simulink library "LinkLayer"  (Simulink 7.4)
settings: Solver=ode45  StartTime=0.0  StopTime=10.0  RelTol=1e-3
settings Model: Creator=dread  LastModifiedBy=dread

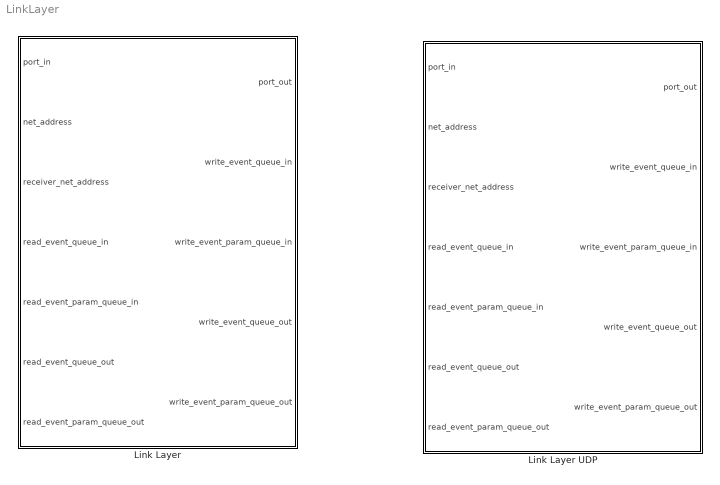
== system LinkLayer ==
  Link Layer : Subsystem  SystemSampleTime=0.1  mask{DelayMin=2, DelayMax=100, MessageLossProbability=0, BufferOverflowPossible=on}
      mask TabNameString: QoS,QoS,QoS,QoS
  Link Layer UDP : Subsystem  SystemSampleTime=0.1  mask{DelayMin=2, DelayMax=100, MessageLossProbability=0}
      mask TabNameString: QoS,QoS,QoS

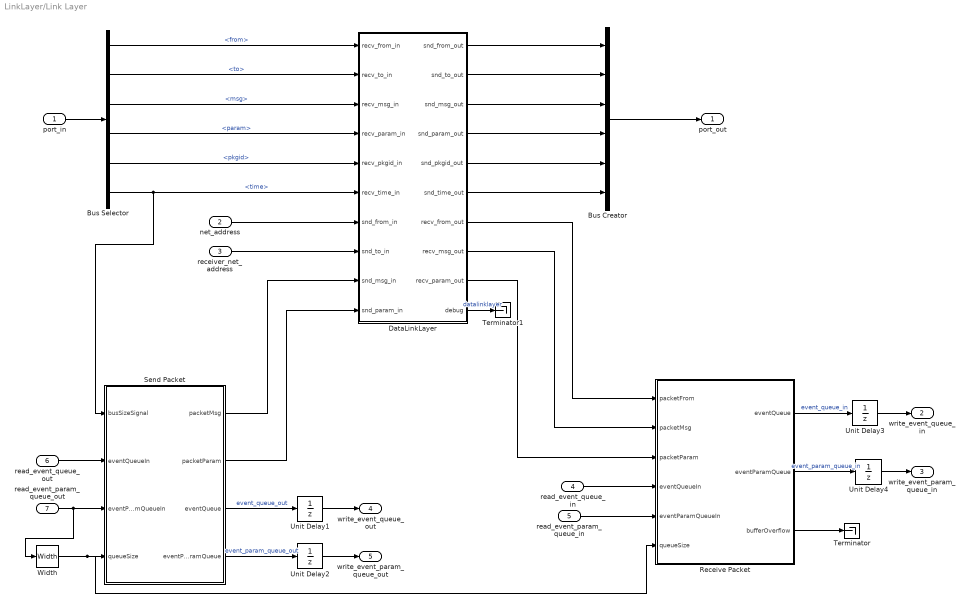
== system LinkLayer/Link Layer ==
  port_in : Inport  UseBusObject=on  OutDataType=fixdt(1, 16)  OutScaling=2^0
      settings: BusObject=PacketBus
  net_address : Inport  Port=2  DataType=uint8  OutDataType=fixdt(1, 16)  OutScaling=2^0  OutDataTypeStr=uint8
  receiver_net_address : Inport  Port=3  DataType=uint8  OutDataType=fixdt(1, 16)  OutScaling=2^0  OutDataTypeStr=uint8
  read_event_queue_in : Inport  Port=4  OutDataType=fixdt(1, 16)  OutScaling=2^0
  read_event_param_queue_in : Inport  Port=5  OutDataType=fixdt(1, 16)  OutScaling=2^0
  read_event_queue_out : Inport  Port=6  OutDataType=fixdt(1, 16)  OutScaling=2^0
  read_event_param_queue_out : Inport  Port=7  OutDataType=fixdt(1, 16)  OutScaling=2^0
  Bus Creator : BusCreator  Inputs=6  UseBusObject=on  NonVirtualBus=on
      settings: BusObject=PacketBus
  Bus Selector : BusSelector  OutputSignals=from,to,msg,param,pkgid,time
  DataLinkLayer : Subsystem
  Receive Packet : Stateflow chart
  Send Packet : Stateflow chart
  Terminator : Terminator
  Terminator1 : Terminator
  Unit Delay{1..4} (4 alike) : UnitDelay  SampleTime=-1
  Width : Width  DataType=uint32
  port_out : Outport  UseBusObject=on  OutDataType=fixdt(1, 16)  OutScaling=2^0
      settings: BusObject=PacketBus
  write_event_queue_in : Outport  Port=2  OutDataType=fixdt(1, 16)  OutScaling=2^0
  write_event_param_queue_in : Outport  Port=3  OutDataType=fixdt(1, 16)  OutScaling=2^0
  write_event_queue_out : Outport  Port=4  OutDataType=fixdt(1, 16)  OutScaling=2^0
  write_event_param_queue_out : Outport  Port=5  OutDataType=fixdt(1, 16)  OutScaling=2^0
  wires:
  Receive Packet/2(eventParamQueue) -> Unit Delay4/1  "event_param_queue_in"
  Receive Packet/1(eventQueue) -> Unit Delay3/1  "event_queue_in"
  Send Packet/4(eventParamQueue) -> Unit Delay2/1  "event_param_queue_out"
  Send Packet/3(eventQueue) -> Unit Delay1/1  "event_queue_out"
  read_event_queue_out/1 -> Send Packet/2(eventQueueIn)
  net_address/1 -> DataLinkLayer/7(snd_from_in)
  Send Packet/1(packetMsg) -> DataLinkLayer/9(snd_msg_in)
  DataLinkLayer/9(recv_param_out) -> Receive Packet/3(packetParam)
  DataLinkLayer/8(recv_msg_out) -> Receive Packet/2(packetMsg)
  DataLinkLayer/7(recv_from_out) -> Receive Packet/1(packetFrom)
  Bus Selector/3 -> DataLinkLayer/3(recv_msg_in)  "<msg>"
  Bus Selector/5 -> DataLinkLayer/5(recv_pkgid_in)  "<pkgid>"
  Bus Selector/6 -> Send Packet/1(busSizeSignal), DataLinkLayer/6(recv_time_in)  "<time>"
  port_in/1 -> Bus Selector/1
  Bus Creator/1 -> port_out/1
  Bus Selector/2 -> DataLinkLayer/2(recv_to_in)  "<to>"
  Bus Selector/1 -> DataLinkLayer/1(recv_from_in)  "<from>"
  Send Packet/2(packetParam) -> DataLinkLayer/10(snd_param_in)
  Bus Selector/4 -> DataLinkLayer/4(recv_param_in)  "<param>"
  read_event_queue_in/1 -> Receive Packet/4(eventQueueIn)
  read_event_param_queue_in/1 -> Receive Packet/5(eventParamQueueIn)
  read_event_param_queue_out/1 -> Send Packet/3(eventParamQueueIn), Width/1
  DataLinkLayer/1(snd_from_out) -> Bus Creator/1
  DataLinkLayer/2(snd_to_out) -> Bus Creator/2
  DataLinkLayer/3(snd_msg_out) -> Bus Creator/3
  DataLinkLayer/4(snd_param_out) -> Bus Creator/4
  DataLinkLayer/5(snd_pkgid_out) -> Bus Creator/5
  DataLinkLayer/6(snd_time_out) -> Bus Creator/6
  Receive Packet/3(bufferOverflow) -> Terminator/1
  Unit Delay1/1 -> write_event_queue_out/1
  Unit Delay2/1 -> write_event_param_queue_out/1
  Unit Delay3/1 -> write_event_queue_in/1
  Unit Delay4/1 -> write_event_param_queue_in/1
  receiver_net_address/1 -> DataLinkLayer/8(snd_to_in)
  Width/1 -> Receive Packet/6(queueSize), Send Packet/4(queueSize)
  DataLinkLayer/10(debug) -> Terminator1/1  "datalinklayer"

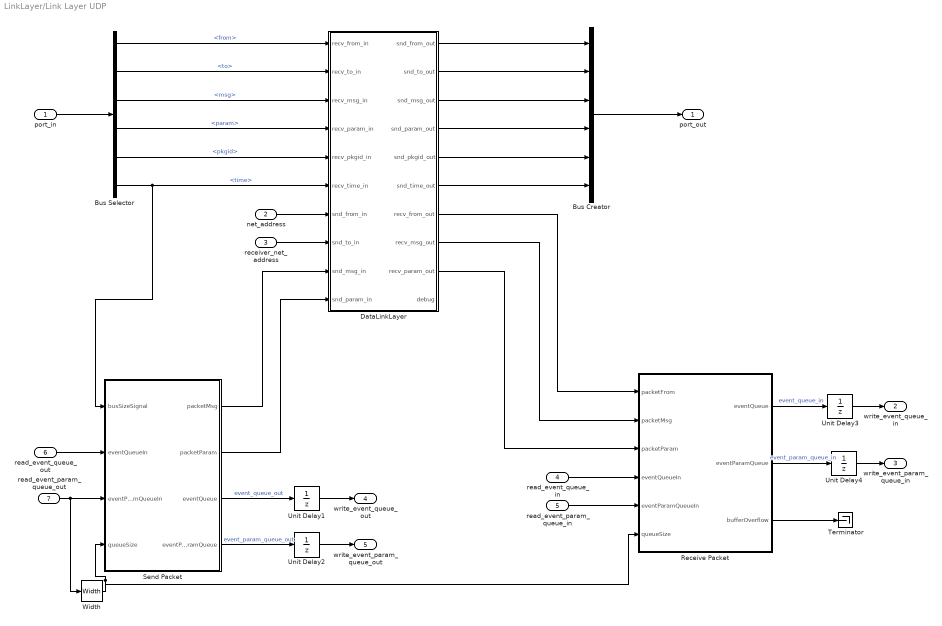
== system LinkLayer/Link Layer UDP ==
  port_in : Inport  UseBusObject=on  OutDataType=fixdt(1, 16)  OutScaling=2^0
      settings: BusObject=PacketBus
  net_address : Inport  Port=2  DataType=uint8  OutDataType=fixdt(1, 16)  OutScaling=2^0  OutDataTypeStr=uint8
  receiver_net_address : Inport  Port=3  DataType=uint8  OutDataType=fixdt(1, 16)  OutScaling=2^0  OutDataTypeStr=uint8
  read_event_queue_in : Inport  Port=4  OutDataType=fixdt(1, 16)  OutScaling=2^0
  read_event_param_queue_in : Inport  Port=5  OutDataType=fixdt(1, 16)  OutScaling=2^0
  read_event_queue_out : Inport  Port=6  OutDataType=fixdt(1, 16)  OutScaling=2^0
  read_event_param_queue_out : Inport  Port=7  OutDataType=fixdt(1, 16)  OutScaling=2^0
  Bus Creator : BusCreator  Inputs=6  UseBusObject=on
      settings: BusObject=PacketBus
  Bus Selector : BusSelector  OutputSignals=from,to,msg,param,pkgid,time
  DataLinkLayer : Subsystem
  Receive Packet : Stateflow chart
  Send Packet : Stateflow chart
  Terminator : Terminator
  Unit Delay{1..4} (4 alike) : UnitDelay  SampleTime=-1
  Width : Width  DataType=uint32
  port_out : Outport  UseBusObject=on  OutDataType=fixdt(1, 16)  OutScaling=2^0
      settings: BusObject=PacketBus
  write_event_queue_in : Outport  Port=2  OutDataType=fixdt(1, 16)  OutScaling=2^0
  write_event_param_queue_in : Outport  Port=3  OutDataType=fixdt(1, 16)  OutScaling=2^0
  write_event_queue_out : Outport  Port=4  OutDataType=fixdt(1, 16)  OutScaling=2^0
  write_event_param_queue_out : Outport  Port=5  OutDataType=fixdt(1, 16)  OutScaling=2^0
  wires:
  net_address/1 -> DataLinkLayer/7(snd_from_in)
  Send Packet/1(packetMsg) -> DataLinkLayer/9(snd_msg_in)
  DataLinkLayer/9(recv_param_out) -> Receive Packet/3(packetParam)
  DataLinkLayer/8(recv_msg_out) -> Receive Packet/2(packetMsg)
  DataLinkLayer/7(recv_from_out) -> Receive Packet/1(packetFrom)
  Bus Selector/3 -> DataLinkLayer/3(recv_msg_in)  "<msg>"
  Bus Selector/5 -> DataLinkLayer/5(recv_pkgid_in)  "<pkgid>"
  Bus Selector/6 -> Send Packet/1(busSizeSignal), DataLinkLayer/6(recv_time_in)  "<time>"
  port_in/1 -> Bus Selector/1
  Bus Creator/1 -> port_out/1
  Bus Selector/2 -> DataLinkLayer/2(recv_to_in)  "<to>"
  Bus Selector/1 -> DataLinkLayer/1(recv_from_in)  "<from>"
  Send Packet/2(packetParam) -> DataLinkLayer/10(snd_param_in)
  Bus Selector/4 -> DataLinkLayer/4(recv_param_in)  "<param>"
  DataLinkLayer/1(snd_from_out) -> Bus Creator/1
  DataLinkLayer/2(snd_to_out) -> Bus Creator/2
  DataLinkLayer/3(snd_msg_out) -> Bus Creator/3
  DataLinkLayer/4(snd_param_out) -> Bus Creator/4
  DataLinkLayer/5(snd_pkgid_out) -> Bus Creator/5
  DataLinkLayer/6(snd_time_out) -> Bus Creator/6
  Receive Packet/2(eventParamQueue) -> Unit Delay4/1  "event_param_queue_in"
  Receive Packet/1(eventQueue) -> Unit Delay3/1  "event_queue_in"
  Unit Delay3/1 -> write_event_queue_in/1
  Unit Delay4/1 -> write_event_param_queue_in/1
  Receive Packet/3(bufferOverflow) -> Terminator/1
  Send Packet/4(eventParamQueue) -> Unit Delay2/1  "event_param_queue_out"
  Send Packet/3(eventQueue) -> Unit Delay1/1  "event_queue_out"
  Unit Delay1/1 -> write_event_queue_out/1
  Unit Delay2/1 -> write_event_param_queue_out/1
  receiver_net_address/1 -> DataLinkLayer/8(snd_to_in)
  read_event_queue_in/1 -> Receive Packet/4(eventQueueIn)
  read_event_param_queue_in/1 -> Receive Packet/5(eventParamQueueIn)
  read_event_queue_out/1 -> Send Packet/2(eventQueueIn)
  read_event_param_queue_out/1 -> Send Packet/3(eventParamQueueIn), Width/1
  Width/1 -> Send Packet/4(queueSize), Receive Packet/6(queueSize)

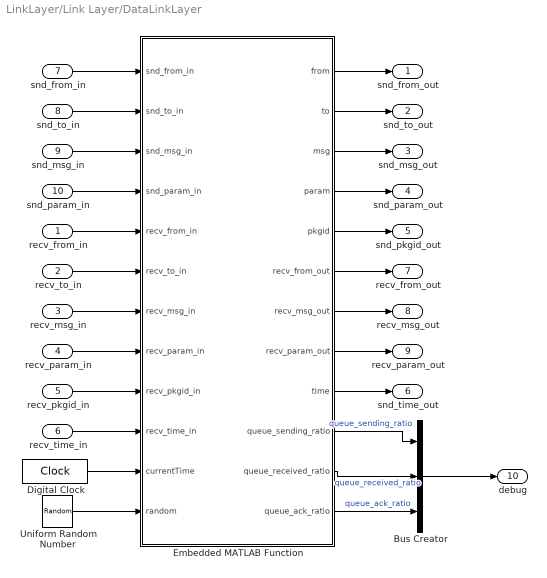
== system LinkLayer/Link Layer/DataLinkLayer ==
  recv_from_in : Inport  DataType=uint8  OutDataType=fixdt(1, 16)  OutScaling=2^0  OutDataTypeStr=uint8
  recv_to_in : Inport  Port=2  DataType=uint8  OutDataType=fixdt(1, 16)  OutScaling=2^0  OutDataTypeStr=uint8
  recv_msg_in : Inport  Port=3  DataType=uint16  OutDataType=fixdt(1, 16)  OutScaling=2^0  OutDataTypeStr=uint16
  recv_param_in : Inport  Port=4  DataType=double  OutDataType=fixdt(1, 16)  OutScaling=2^0  OutDataTypeStr=double
  recv_pkgid_in : Inport  Port=5  DataType=uint32  OutDataType=fixdt(1, 16)  OutScaling=2^0  OutDataTypeStr=uint32
  recv_time_in : Inport  Port=6  DataType=double  OutDataType=fixdt(1, 16)  OutScaling=2^0  OutDataTypeStr=double
  snd_from_in : Inport  Port=7  DataType=uint8  OutDataType=fixdt(1, 16)  OutScaling=2^0  OutDataTypeStr=uint8
  snd_to_in : Inport  Port=8  DataType=uint8  OutDataType=fixdt(1, 16)  OutScaling=2^0  OutDataTypeStr=uint8
  snd_msg_in : Inport  Port=9  DataType=uint16  OutDataType=fixdt(1, 16)  OutScaling=2^0  OutDataTypeStr=uint16
  snd_param_in : Inport  Port=10  DataType=double  OutDataType=fixdt(1, 16)  OutScaling=2^0  OutDataTypeStr=double
  Bus Creator : BusCreator  Inputs=3
  Digital Clock : DigitalClock  SampleTime=0.001
  Embedded MATLAB Function : Stateflow chart  TreatAsAtomicUnit=on
  Uniform Random Number : UniformRandomNumber  Minimum=0  Maximum=100  SampleTime=0.001
  snd_from_out : Outport  DataType=uint8  OutDataType=fixdt(1, 16)  OutScaling=2^0  OutDataTypeStr=uint8
  snd_to_out : Outport  Port=2  DataType=uint8  OutDataType=fixdt(1, 16)  OutScaling=2^0  OutDataTypeStr=uint8
  snd_msg_out : Outport  Port=3  DataType=uint16  OutDataType=fixdt(1, 16)  OutScaling=2^0  OutDataTypeStr=uint16
  snd_param_out : Outport  Port=4  DataType=double  OutDataType=fixdt(1, 16)  OutScaling=2^0  OutDataTypeStr=double
  snd_pkgid_out : Outport  Port=5  DataType=uint32  OutDataType=fixdt(1, 16)  OutScaling=2^0  OutDataTypeStr=uint32
  snd_time_out : Outport  Port=6  DataType=double  OutDataType=fixdt(1, 16)  OutScaling=2^0  OutDataTypeStr=double
  recv_from_out : Outport  Port=7  DataType=uint8  OutDataType=fixdt(1, 16)  OutScaling=2^0  OutDataTypeStr=uint8
  recv_msg_out : Outport  Port=8  DataType=uint16  OutDataType=fixdt(1, 16)  OutScaling=2^0  OutDataTypeStr=uint16
  recv_param_out : Outport  Port=9  DataType=double  OutDataType=fixdt(1, 16)  OutScaling=2^0  OutDataTypeStr=double
  debug : Outport  Port=10  OutDataType=fixdt(1, 16)  OutScaling=2^0
  wires:
  Embedded MATLAB Function/9(time) -> snd_time_out/1
  recv_time_in/1 -> Embedded MATLAB Function/10(recv_time_in)
  recv_pkgid_in/1 -> Embedded MATLAB Function/9(recv_pkgid_in)
  recv_param_in/1 -> Embedded MATLAB Function/8(recv_param_in)
  recv_msg_in/1 -> Embedded MATLAB Function/7(recv_msg_in)
  recv_to_in/1 -> Embedded MATLAB Function/6(recv_to_in)
  recv_from_in/1 -> Embedded MATLAB Function/5(recv_from_in)
  Embedded MATLAB Function/8(recv_param_out) -> recv_param_out/1
  Embedded MATLAB Function/7(recv_msg_out) -> recv_msg_out/1
  Embedded MATLAB Function/6(recv_from_out) -> recv_from_out/1
  snd_to_in/1 -> Embedded MATLAB Function/2(snd_to_in)
  snd_from_in/1 -> Embedded MATLAB Function/1(snd_from_in)
  snd_param_in/1 -> Embedded MATLAB Function/4(snd_param_in)
  snd_msg_in/1 -> Embedded MATLAB Function/3(snd_msg_in)
  Embedded MATLAB Function/5(pkgid) -> snd_pkgid_out/1
  Embedded MATLAB Function/4(param) -> snd_param_out/1
  Embedded MATLAB Function/3(msg) -> snd_msg_out/1
  Embedded MATLAB Function/2(to) -> snd_to_out/1
  Embedded MATLAB Function/1(from) -> snd_from_out/1
  Bus Creator/1 -> debug/1
  Embedded MATLAB Function/10(queue_sending_ratio) -> Bus Creator/1  "queue_sending_ratio"
  Embedded MATLAB Function/11(queue_received_ratio) -> Bus Creator/2  "queue_received_ratio"
  Embedded MATLAB Function/12(queue_ack_ratio) -> Bus Creator/3  "queue_ack_ratio"
  Digital Clock/1 -> Embedded MATLAB Function/11(currentTime)
  Uniform Random Number/1 -> Embedded MATLAB Function/12(random)

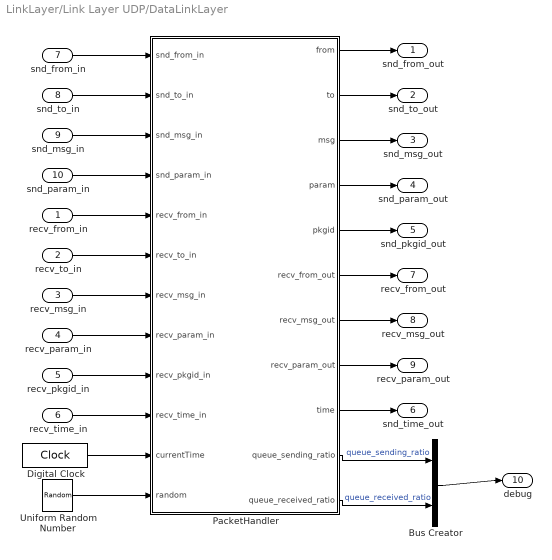
== system LinkLayer/Link Layer UDP/DataLinkLayer ==
  recv_from_in : Inport  DataType=uint8  OutDataType=fixdt(1, 16)  OutScaling=2^0  OutDataTypeStr=uint8
  recv_to_in : Inport  Port=2  DataType=uint8  OutDataType=fixdt(1, 16)  OutScaling=2^0  OutDataTypeStr=uint8
  recv_msg_in : Inport  Port=3  DataType=uint16  OutDataType=fixdt(1, 16)  OutScaling=2^0  OutDataTypeStr=uint16
  recv_param_in : Inport  Port=4  DataType=double  OutDataType=fixdt(1, 16)  OutScaling=2^0  OutDataTypeStr=double
  recv_pkgid_in : Inport  Port=5  DataType=uint32  OutDataType=fixdt(1, 16)  OutScaling=2^0  OutDataTypeStr=uint32
  recv_time_in : Inport  Port=6  DataType=double  OutDataType=fixdt(1, 16)  OutScaling=2^0  OutDataTypeStr=double
  snd_from_in : Inport  Port=7  DataType=uint8  OutDataType=fixdt(1, 16)  OutScaling=2^0  OutDataTypeStr=uint8
  snd_to_in : Inport  Port=8  DataType=uint8  OutDataType=fixdt(1, 16)  OutScaling=2^0  OutDataTypeStr=uint8
  snd_msg_in : Inport  Port=9  DataType=uint16  OutDataType=fixdt(1, 16)  OutScaling=2^0  OutDataTypeStr=uint16
  snd_param_in : Inport  Port=10  DataType=double  OutDataType=fixdt(1, 16)  OutScaling=2^0  OutDataTypeStr=double
  Bus Creator : BusCreator  Inputs=2
  Digital Clock : DigitalClock  SampleTime=-1
  PacketHandler : Stateflow chart  TreatAsAtomicUnit=on
  Uniform Random Number : UniformRandomNumber  Minimum=0  Maximum=100  SampleTime=0.001
  snd_from_out : Outport  DataType=uint8  OutDataType=fixdt(1, 16)  OutScaling=2^0  OutDataTypeStr=uint8
  snd_to_out : Outport  Port=2  DataType=uint8  OutDataType=fixdt(1, 16)  OutScaling=2^0  OutDataTypeStr=uint8
  snd_msg_out : Outport  Port=3  DataType=uint16  OutDataType=fixdt(1, 16)  OutScaling=2^0  OutDataTypeStr=uint16
  snd_param_out : Outport  Port=4  DataType=double  OutDataType=fixdt(1, 16)  OutScaling=2^0  OutDataTypeStr=double
  snd_pkgid_out : Outport  Port=5  DataType=uint32  OutDataType=fixdt(1, 16)  OutScaling=2^0  OutDataTypeStr=uint32
  snd_time_out : Outport  Port=6  DataType=double  OutDataType=fixdt(1, 16)  OutScaling=2^0  OutDataTypeStr=double
  recv_from_out : Outport  Port=7  DataType=uint8  OutDataType=fixdt(1, 16)  OutScaling=2^0  OutDataTypeStr=uint8
  recv_msg_out : Outport  Port=8  DataType=uint16  OutDataType=fixdt(1, 16)  OutScaling=2^0  OutDataTypeStr=uint16
  recv_param_out : Outport  Port=9  DataType=double  OutDataType=fixdt(1, 16)  OutScaling=2^0  OutDataTypeStr=double
  debug : Outport  Port=10  OutDataType=fixdt(1, 16)  OutScaling=2^0
  wires:
  PacketHandler/9(time) -> snd_time_out/1
  recv_time_in/1 -> PacketHandler/10(recv_time_in)
  recv_pkgid_in/1 -> PacketHandler/9(recv_pkgid_in)
  recv_param_in/1 -> PacketHandler/8(recv_param_in)
  recv_msg_in/1 -> PacketHandler/7(recv_msg_in)
  recv_to_in/1 -> PacketHandler/6(recv_to_in)
  recv_from_in/1 -> PacketHandler/5(recv_from_in)
  PacketHandler/8(recv_param_out) -> recv_param_out/1
  PacketHandler/7(recv_msg_out) -> recv_msg_out/1
  PacketHandler/6(recv_from_out) -> recv_from_out/1
  snd_to_in/1 -> PacketHandler/2(snd_to_in)
  snd_from_in/1 -> PacketHandler/1(snd_from_in)
  snd_param_in/1 -> PacketHandler/4(snd_param_in)
  snd_msg_in/1 -> PacketHandler/3(snd_msg_in)
  PacketHandler/5(pkgid) -> snd_pkgid_out/1
  PacketHandler/4(param) -> snd_param_out/1
  PacketHandler/3(msg) -> snd_msg_out/1
  PacketHandler/2(to) -> snd_to_out/1
  PacketHandler/1(from) -> snd_from_out/1
  Bus Creator/1 -> debug/1
  PacketHandler/10(queue_sending_ratio) -> Bus Creator/1  "queue_sending_ratio"
  PacketHandler/11(queue_received_ratio) -> Bus Creator/2  "queue_received_ratio"
  Digital Clock/1 -> PacketHandler/11(currentTime)
  Uniform Random Number/1 -> PacketHandler/12(random)

== matlab function Link Layer/Receive Packet ==
  settings: updateMethod=DISCRETE  sampleTime=0.001
  data: packetFrom input double; packetMsg input double; packetParam input double; eventQueueIn input uint8; eventParamQueueIn input double; eventQueue output uint8; eventParamQueue output double; bufferOverflow output boolean; queueSize input uint32
function [eventQueue, eventParamQueue, bufferOverflow] = receivePacket(packetFrom, packetMsg, packetParam, eventQueueIn, eventParamQueueIn, queueSize)
%#eml
% This function receives packets and adds them to the event queue.
% A packet consists of a source, a message and an optional parameter for 
% the message. Source and message are contained at position 1 and 2 in the 
% eventQueue. Because of the different data type the parameter has his own 
% queue eventParamQueue.

%Constants
SOURCE = 2;
MESSAGE = 1;
BUS_SIZE = numel(packetFrom);
QUEUE_SIZE = queueSize;

%Init
eventQueue = eventQueueIn;
eventParamQueue = eventParamQueueIn;
bufferOverflow = false;

%New incoming packet
for i = 1:BUS_SIZE
    if packetFrom(i) ~= 0 
        bufferOverflow = true;
        %Add it to the incoming event Queue
        for j = 1:QUEUE_SIZE
            %Search for an empty place
            if eventQueue(j,SOURCE) == 0
                eventQueue(j,SOURCE)    = packetFrom(i);
                eventQueue(j,MESSAGE)   = packetMsg(i);
                eventParamQueue(j)      = packetParam(i);
                bufferOverflow = false;
                break;
            end
        end        
    else
        break;
    end
end

== matlab function Link Layer/Send Packet ==
  settings: updateMethod=DISCRETE  sampleTime=0.001
  data: busSizeSignal input double; packetMsg output double; packetParam output double; eventQueue output uint8; eventParamQueue output double; eventQueueIn input uint8; eventParamQueueIn input double; queueSize input uint32
function [packetMsg, packetParam, eventQueue, eventParamQueue] = sendPacket(busSizeSignal, eventQueueIn, eventParamQueueIn, queueSize)
%#eml

% This function creates packets from the event queue. A packet consists
% of a destination, a message and an optional parameter for the message.
% Destination and message are contained at position 1 and 2 in the 
% eventQueue. Because of the different data type the parameter has his own 
% queue eventParamQueue.

%Constants
DESTINATION = 2;
MESSAGE = 1;
QUEUE_SIZE = queueSize;

busSize = numel(busSizeSignal);

%Init
eventQueue = eventQueueIn;
eventParamQueue = eventParamQueueIn;
packetMsg = zeros(1,busSize,'uint16');
packetParam = zeros(1,busSize,'double');

%There is an event in the queue
for i = 1:busSize   
    if eventQueue(1,DESTINATION) ~= 0 || eventQueue(1,MESSAGE) ~= 0
        %Create packet from the firs entry in the queue
        packetMsg(i)   = uint16(eventQueue(1,MESSAGE));
        packetParam(i) = eventParamQueue(1);
        %Remove the event from the queue
        for j=1:QUEUE_SIZE - 1
            eventQueue(j,DESTINATION)   = eventQueue(j+1,DESTINATION);
            eventQueue(j,MESSAGE)       = eventQueue(j+1,MESSAGE);
            eventParamQueue(j)          = eventParamQueue(j+1);
        end
        %Set last element to zero
        eventQueue(QUEUE_SIZE,DESTINATION)  = 0;
        eventQueue(QUEUE_SIZE,MESSAGE)      = 0;
        eventParamQueue(QUEUE_SIZE)    = 0;
    else
        break;
    end
end

== matlab function Link Layer UDP/DataLinkLayer/PacketHandler ==
  settings: updateMethod=DISCRETE
  data: snd_from_in input double; snd_to_in input double; snd_msg_in input double; snd_param_in input double; from output double; to output double; msg output double; param output double; pkgid output double; recv_from_in input double; recv_to_in input double; recv_msg_in input double; recv_param_in input double; recv_pkgid_in input uint32; recv_from_out output double; recv_msg_out output double; recv_param_out output double; recv_time_in input double; time output double; currentTime input double; queue_sending_ratio output double; queue_received_ratio output double; DelayMin parameter uint32; DelayMax parameter uint32; MessageLossProbability parameter uint32; random input double
function [from, to, msg, param, pkgid, recv_from_out, recv_msg_out, recv_param_out, time, queue_sending_ratio, queue_received_ratio] = packetHandler(snd_from_in, snd_to_in, snd_msg_in, snd_param_in, recv_from_in, recv_to_in, recv_msg_in, recv_param_in, recv_pkgid_in, recv_time_in, currentTime, DelayMin, DelayMax, MessageLossProbability, random)
%#eml
eml.extrinsic('warning', 'disp', 'fprintf');

%Constants
BUS_SIZE =  1;%numel(snd_from_in);
QUEUE_SIZE_SENDING = 10 * BUS_SIZE;
QUEUE_SIZE_RECEIVED = 10 *BUS_SIZE;
SAMPLE_TIME = 0.001;
PHYSICAL_DELAY = 2;

%Constraints
if DelayMin < 2
    DelayMin = uint32(2);
end

%Time to delay each outgoing packet
assert(DelayMin >= PHYSICAL_DELAY);
delay_time =  double(DelayMin - PHYSICAL_DELAY) * SAMPLE_TIME;

%Init
from    = zeros(1,BUS_SIZE,'uint8');
to      = zeros(1,BUS_SIZE,'uint8');
msg     = zeros(1,BUS_SIZE,'uint16');
param   = zeros(1,BUS_SIZE,'double');
pkgid   = zeros(1,BUS_SIZE,'uint32');
time    = zeros(1,BUS_SIZE,'double');
 
recv_from_out    = zeros(1,BUS_SIZE,'uint8');
recv_msg_out     = zeros(1,BUS_SIZE,'uint16');
recv_param_out   = zeros(1,BUS_SIZE,'double');


recv_in = bus(recv_from_in, recv_to_in, recv_msg_in, recv_param_in, recv_pkgid_in, recv_time_in, BUS_SIZE);



%Persistent variables
persistent sendingQueue receivedQueue lastPkgid

if isempty(lastPkgid)
    lastPkgid = uint32(0);
end

if isempty(sendingQueue)
    sendingQueue = repmat(packet(0,0,0,0,0,0), 1, QUEUE_SIZE_SENDING);
end


if isempty(receivedQueue)
    receivedQueue = repmat(packet(0, 0, 0, 0, 0, 0), 1, QUEUE_SIZE_RECEIVED);
end

%compute stats
queue_sending_ratio = queueNumElements(sendingQueue)/QUEUE_SIZE_SENDING;
queue_received_ratio = queueNumElements(receivedQueue)/QUEUE_SIZE_RECEIVED;

%Step 1: Check for a new outgoing packet
for i = 1:BUS_SIZE    
    if snd_msg_in(i) ~= 0
        lastPkgid = lastPkgid +1;
        outgoing = packet(snd_from_in, snd_to_in(i), snd_msg_in(i), snd_param_in(i), lastPkgid, currentTime);

        %Add packet so the outgoing queue
        sendingQueue = enqueue(sendingQueue, outgoing); 
    end
end
    
%Step 2: Check for a new incoming packet
for i = 1:length(recv_in)
    incoming = packet(recv_in(i).from, recv_in(i).to, recv_in(i).msg, recv_in(i).param, recv_in(i).pkgid, recv_in(i).time);
    if incoming.from ~= 0 && incoming.to == snd_from_in && ~dropPacket(incoming, MessageLossProbability, random)
        
        %Check if max_delay is valid
        if incoming.time + (double(DelayMax) * SAMPLE_TIME) < currentTime
            %Exceeded max delay. Drop packet.
            continue;
        end

        %save packet
        receivedQueue = enqueue(receivedQueue, incoming); 
    end
end

%Step 3: Forward incoming packet
for i = 1:BUS_SIZE
    if receivedQueue(1).from ~= 0
        recv_from_out(i)    = receivedQueue(1).from;
        recv_msg_out(i)     = receivedQueue(1).msg;
        recv_param_out(i)   = receivedQueue(1).param;
        receivedQueue = dequeue(receivedQueue,1);
    else
        break;
    end
end


%Step 4: Send outgoing packet
for i = 1:BUS_SIZE
    if sendingQueue(1).to ~= 0  && minDelayExpired(sendingQueue(1), currentTime, delay_time) %Respect minimum delay
        from(i)    = sendingQueue(1).from;
        to(i)      = sendingQueue(1).to;
        msg(i)     = sendingQueue(1).msg;
        param(i)   = sendingQueue(1).param;
        pkgid(i)   = sendingQueue(1).pkgid;
        time(i)    = sendingQueue(1).time;

        %remove packet from sending queue
        sendingQueue = dequeue(sendingQueue, 1);    
    else
        break;
    end
end


%%%%%%%%%%%%%%%%%%%%%%%%%%%%%%%%%%%%%%%%%%%%%%%%%%%%%%%%%%%%%%%%%%%%%%%%%%%
%%                          H E L P E R
%%%%%%%%%%%%%%%%%%%%%%%%%%%%%%%%%%%%%%%%%%%%%%%%%%%%%%%%%%%%%%%%%%%%%%%%%%%

function p = packet(from, to, msg, param, pkgid, time)
%#eml
%Defines a packet
p = struct('from', uint8(from),'to', uint8(to),'msg', uint16(msg),'param', double(param),'pkgid', uint32(pkgid), 'time', double(time));

function bus = bus(from, to, msg, param, pkgid, time, size) %emp
%Create an empty bus
bus = repmat(packet(0,0,0,0,0,0), 1, size);
for i=1:size
    bus(i) = packet(from(i), to(i), msg(i), param(i), pkgid(i), time(i));
end


function queue = enqueue(queue, packet)
%#eml
eml.extrinsic('warning', 'sprintf');
for i = 1:length(queue)
    if queue(i).to == 0
        queue(i) = packet;
        return;
    end
end
warning('DataLinkLayer:enqueue', 'DataLinkLayer Buffer overflow. Dropping packet  %3u: %u->%u :%3u (%.1f) @%.2f', packet.pkgid, packet.from, packet.to, packet.msg, packet.param, packet.time);

function queue = dequeue(queue, index)
%#eml
assert(index <= length(queue))
for i=index:length(queue)-1;
    queue(i) = queue(i+1);
end
queue(length(queue)) = packet(0,0,0,0,0,0);

function num = queueNumElements(queue)
%#eml
num = 0;
for i = 1:length(queue)
    if queue(i).to ~= uint8(0)
        num = num+1;
    end
end    

function packetString = toString(packet) %#eml
eml.extrinsic('sprintf');
packetString = sprintf('%3u: %u->%u :%3u (%.2f) @%.3f', packet.pkgid, packet.from, packet.to, packet.msg, packet.param, packet.time);

%Wheter the packet is ready to fire or not.
function expired = minDelayExpired(packet, current_time, delay_time) %eml
eml.extrinsic('warning');
expired = (packet.time + delay_time) <= current_time;

%Drop message with a given probability
function drop = dropPacket(p, probability, random) %eml
drop = random < probability;

== matlab function Link Layer/DataLinkLayer/Embedded MATLAB Function ==
  settings: updateMethod=DISCRETE  sampleTime=0.001
  data: snd_from_in input double; snd_to_in input double; snd_msg_in input double; snd_param_in input double; from output double; to output double; msg output double; param output double; pkgid output double; recv_from_in input double; recv_to_in input double; recv_msg_in input double; recv_param_in input double; recv_pkgid_in input uint32; recv_from_out output double; recv_msg_out output double; recv_param_out output double; recv_time_in input double; time output double; currentTime input double; queue_sending_ratio output double; queue_received_ratio output double; queue_ack_ratio output double; DelayMin parameter uint32; DelayMax parameter uint32; BufferOverflowPossible parameter boolean; MessageLossProbability parameter uint32; random input double
function [from, to, msg, param, pkgid, recv_from_out, recv_msg_out, recv_param_out, time, queue_sending_ratio, queue_received_ratio, queue_ack_ratio] = ackHandler(snd_from_in, snd_to_in, snd_msg_in, snd_param_in, recv_from_in, recv_to_in, recv_msg_in, recv_param_in, recv_pkgid_in, recv_time_in, currentTime, DelayMin, DelayMax, BufferOverflowPossible, MessageLossProbability, random)
%#eml
eml.extrinsic('warning', 'disp', 'fprintf', 'error');

%Constants
SAMPLE_TIME = 0.001;
BUS_SIZE =  numel(snd_msg_in);
MSG_ACK         = 255;
QUEUE_SIZE_SENDING = 10 * BUS_SIZE;
QUEUE_SIZE_ACK  = 10* BUS_SIZE;
QUEUE_SIZE_RECEIVED = 10 *BUS_SIZE;
QUEUE_SIZE_INORDER = 10* BUS_SIZE;

PHYSICAL_DELAY = 2;

%Constraints
if DelayMin < PHYSICAL_DELAY
    DelayMin = uint32(PHYSICAL_DELAY);
end

DELAY_MIN_TIME = double(DelayMin) * SAMPLE_TIME;
DELAY_MAX_TIME = double(DelayMax) * SAMPLE_TIME;


%Time to wait for an ACK
TIMEOUT_ACK = DELAY_MIN_TIME * 4.0;

%Time to delay each outgoing packet
assert(DelayMin >= PHYSICAL_DELAY);
delay_time =  double(DelayMin - PHYSICAL_DELAY) * SAMPLE_TIME;



%Init
from    = zeros(1,BUS_SIZE,'uint8');
to      = zeros(1,BUS_SIZE,'uint8');
msg     = zeros(1,BUS_SIZE,'uint16');
param   = zeros(1,BUS_SIZE,'double');
pkgid   = zeros(1,BUS_SIZE,'uint32');
time    = zeros(1,BUS_SIZE,'double');
 
recv_from_out    = zeros(1,BUS_SIZE,'uint8');
recv_msg_out     = zeros(1,BUS_SIZE,'uint16');
recv_param_out   = zeros(1,BUS_SIZE,'double');


recv_in = bus(recv_from_in, recv_to_in, recv_msg_in, recv_param_in, recv_pkgid_in, recv_time_in, BUS_SIZE);



%Persistent variables
persistent sendingQueue ackQueue receivedQueue lastPkgid expectPkgid expectTime inOrderQueue

if isempty(lastPkgid)
    lastPkgid = uint32(0);
end

%The next packet id that we are expecting
if isempty(expectPkgid)
    expectPkgid = uint32(1);
end

%The time we detected a packet loss
if isempty(expectTime)
    expectTime = currentTime;
end


if isempty(sendingQueue)
    sendingQueue = repmat(packet(0,0,0,0,0,0), 1, QUEUE_SIZE_SENDING);
end

if isempty(ackQueue)
    ackQueue = repmat(packet(0,0,0,0,0,0), 1, QUEUE_SIZE_ACK);
end

if isempty(receivedQueue)
    receivedQueue = repmat(packet(0, 0, 0, 0, 0, 0), 1, QUEUE_SIZE_RECEIVED);
end

%Queue to ensure packets are received in order
if isempty(inOrderQueue)
    inOrderQueue = repmat(packet(0, 0, 0, 0, 0, 0), 1, QUEUE_SIZE_INORDER);
end

%compute stats
queue_sending_ratio = queueNumElements(sendingQueue)/QUEUE_SIZE_SENDING;
queue_ack_ratio = queueNumElements(ackQueue)/QUEUE_SIZE_ACK;
queue_received_ratio = queueNumElements(receivedQueue)/QUEUE_SIZE_RECEIVED;

%Step 1: Check for a new outgoing packet
for i = 1:BUS_SIZE    
    if snd_msg_in(i) ~= 0
        lastPkgid = lastPkgid +1;
        outgoing = packet(snd_from_in, snd_to_in, snd_msg_in(i), snd_param_in(i), lastPkgid, currentTime);

        %Add packet so the outgoing queue
        sendingQueue = enqueue(sendingQueue, outgoing, BufferOverflowPossible); 
    end
end
    
%Step 2: Check for a new incoming packet
for i = 1:length(recv_in)
    incoming = packet(recv_in(i).from, recv_in(i).to, recv_in(i).msg, recv_in(i).param, recv_in(i).pkgid, recv_in(i).time);
    if incoming.from ~= 0 && incoming.to == snd_from_in && ~dropPacket(incoming, MessageLossProbability, random)
        
        %Check if message is in delay range
        if incoming.time + DELAY_MAX_TIME < currentTime
            %Exceeded max delay. Drop packet.
            continue;
        end
        
        if incoming.msg == MSG_ACK
            %Remove packet from ackQueue
            for j=1:length(ackQueue)
                if ackQueue(j).pkgid == uint32(incoming.param)
                    ackQueue = dequeue(ackQueue,j);
                end
            end
        else
            %Send ACK
            ackPacket = packet(incoming.to, incoming.from, MSG_ACK, double(incoming.pkgid),incoming.pkgid, currentTime);
            sendingQueue = enqueue(sendingQueue, ackPacket, BufferOverflowPossible);

           %Drop all packets we've already received
           if incoming.pkgid < expectPkgid
               warning('LinkLayer:incomingPacket', 'Dropping late packet %s', toString(incoming));               
           %Accept the packet we are waiting for
           elseif incoming.pkgid == expectPkgid
               receivedQueue = enqueue(receivedQueue, incoming, BufferOverflowPossible);
               expectPkgid = expectPkgid + 1;               
           %Packet loss detected! Save the packet for later processing. 
           else %incoming.pkgid > expectedPkgid       
               % We are not yet waiting for a packet. Set the timeout.
               if queueNumElements(inOrderQueue) == 0 
                   expectTime = currentTime;
                   warning('LinkLayer:incomingPacket', 'Packet loss detected. Waiting for %u', expectPkgid);
               end
               inOrderQueue = enqueue(inOrderQueue, incoming, BufferOverflowPossible);               
           end
           
        end
    end
end

%Step 3: Check if we can process packets from the inorder queue
if queueNumElements(inOrderQueue) > 0
    
    %Did we reach a timeout?
    if expectTime + DELAY_MAX_TIME < currentTime
        warning('LinkLayer:incomingPacket', 'Timeout reached waiting for %u. Dropping packet. Processing queue.', expectPkgid);
        expectPkgid = expectPkgid + 1;    
        expectTime = currentTime;
    end
    
   %Check if we have the expectPkgid in the queue
   foundNext = true;
   while foundNext == true
       foundNext = false;
       for j = 1:length(inOrderQueue)
           if inOrderQueue(j).pkgid == expectPkgid
               %Forward enqueued packet to the received queue
               receivedQueue = enqueue(receivedQueue, inOrderQueue(j), BufferOverflowPossible);                               
               inOrderQueue = dequeue(inOrderQueue, j);
               expectPkgid = expectPkgid + 1;
               foundNext = true;
           elseif inOrderQueue(j).pkgid == 0               
               break;
           end       
       end
   end
end

%Step 4: Forward incoming packet
for i = 1:BUS_SIZE
    if receivedQueue(1).from ~= 0
        recv_from_out(i)    = receivedQueue(1).from;
        recv_msg_out(i)     = receivedQueue(1).msg;
        recv_param_out(i)   = receivedQueue(1).param;
        receivedQueue = dequeue(receivedQueue,1);
    else
        break;
    end
end

%Step 5: ACK timeout reached? Send packet again
for i = 1:length(ackQueue)
    if ackQueue(i).to ~= 0
        if ackQueue(i).acktime + TIMEOUT_ACK <= currentTime
            
            %Update counter
            ackQueue(i).acktime = ackQueue(i).acktime + TIMEOUT_ACK;
            
            %Send again
            if ackQueue(i).acktime + DELAY_MIN_TIME  <= ackQueue(i).time + DELAY_MAX_TIME 
                sendingQueue = enqueue(sendingQueue, ackQueue(i), BufferOverflowPossible);
            else
                warning('LinkLayer:outgoingPacket', 'Timeout reached sending packet %s. Dropping packet.', toString(ackQueue(i)));
            end
            
            %Remove packet from ackQueue
            ackQueue = dequeue(ackQueue, i);
        end
    end
end


%Step 6: Send outgoing packet
for i = 1:BUS_SIZE
    if sendingQueue(1).to ~= 0 && minDelayExpired(sendingQueue(1), currentTime, delay_time) %Respect minimum delay
        from(i)    = sendingQueue(1).from;
        to(i)      = sendingQueue(1).to;
        msg(i)     = sendingQueue(1).msg;
        param(i)   = sendingQueue(1).param;
        pkgid(i)   = sendingQueue(1).pkgid;
        time(i)    = sendingQueue(1).time;

        %Add it to the ack queue
        if sendingQueue(1).msg ~= MSG_ACK
            ackQueue = enqueue(ackQueue, sendingQueue(1), BufferOverflowPossible);
        end

        %remove packet from sending queue
        sendingQueue = dequeue(sendingQueue, 1);    
    else
        break;
    end
end


%%%%%%%%%%%%%%%%%%%%%%%%%%%%%%%%%%%%%%%%%%%%%%%%%%%%%%%%%%%%%%%%%%%%%%%%%%%
%%                          H E L P E R
%%%%%%%%%%%%%%%%%%%%%%%%%%%%%%%%%%%%%%%%%%%%%%%%%%%%%%%%%%%%%%%%%%%%%%%%%%%

function p = packet(from, to, msg, param, pkgid, time)
%#eml
%Defines a packet
p = struct('from', uint8(from),'to', uint8(to),'msg', uint16(msg),'param', double(param),'pkgid', uint32(pkgid), 'time', double(time), 'acktime', double(time));

function bus = bus(from, to, msg, param, pkgid, time, size) %emp
%Create an empty bus
bus = repmat(packet(0,0,0,0,0,0), 1, size);
for i=1:size
    bus(i) = packet(from(i), to(i), msg(i), param(i), pkgid(i), time(i));
end


function queue = enqueue(queue, packet, overflow_allowed)
%#eml
eml.extrinsic('error');
for i = 1:length(queue)
    if queue(i).to == 0
        queue(i) = packet;
        return;
    end
end
if overflow_allowed == false
    error('LinkLayer:DataLinkLayer', 'LinkLayer Buffer overflow. Dropping packet  %s', toString(packet));
end

function queue = dequeue(queue, index)
%#eml
assert(index <= length(queue))
for i=index:length(queue)-1;
    queue(i) = queue(i+1);
end
queue(length(queue)) = packet(0,0,0,0,0,0);

function num = queueNumElements(queue)
%#eml
num = 0;
for i = 1:length(queue)
    if queue(i).to ~= uint8(0)
        num = num+1;
    end
end    

function packetString = toString(packet) %#eml
eml.extrinsic('sprintf');
packetString = sprintf('%3u: %u->%u :%3u (%.2f) @%.4f', packet.pkgid, packet.from, packet.to, packet.msg, packet.param, packet.time);

%Wheter the packet is ready to fire or not.
function expired = minDelayExpired(packet, current_time, delay_time) %eml
eml.extrinsic('warning');
expired = (packet.time + delay_time) <= current_time;

%Drop message with a given probability
function drop = dropPacket(p, probability, random) %eml
drop = random < probability;

== matlab function Link Layer UDP/Receive Packet ==
  settings: updateMethod=DISCRETE
  data: packetFrom input double; packetMsg input double; packetParam input double; eventQueueIn input uint8; eventParamQueueIn input double; queueSize input uint32; eventQueue output uint8; eventParamQueue output double; bufferOverflow output boolean
function [eventQueue, eventParamQueue, bufferOverflow] = receivePacket(packetFrom, packetMsg, packetParam, eventQueueIn, eventParamQueueIn, queueSize)
%#eml
% This function receives packets and adds them to the event queue.
% A packet consists of a source, a message and an optional parameter for 
% the message. Source and message are contained at position 1 and 2 in the 
% eventQueue. Because of the different data type the parameter has his own 
% queue eventParamQueue.
eml.extrinsic('fprintf');
%Constants
SOURCE = 2;
MESSAGE = 1;
BUS_SIZE = numel(packetFrom);
QUEUE_SIZE = queueSize;

%Init
eventQueue = eventQueueIn;
eventParamQueue = eventParamQueueIn;
bufferOverflow = false;

%New incoming packet
for i = 1:BUS_SIZE
    if packetFrom(i) ~= 0 
        bufferOverflow = true;
        %Add it to the incoming event Queue
        for j = 1:QUEUE_SIZE
            %Search for an empty place
            if eventQueue(j,SOURCE) == 0
                eventQueue(j,SOURCE)    = packetFrom(i);
                eventQueue(j,MESSAGE)   = packetMsg(i);
                eventParamQueue(j)      = packetParam(i);
                bufferOverflow = false;
                break;
            end
        end
    else
        break;
    end
end

== matlab function Link Layer UDP/Send Packet ==
  settings: updateMethod=DISCRETE
  data: busSizeSignal input double; packetMsg output double; packetParam output double; eventQueue output uint8; eventParamQueue output double; eventQueueIn input uint8; eventParamQueueIn input double; queueSize input uint32
function [packetMsg, packetParam, eventQueue, eventParamQueue] = sendPacket(busSizeSignal, eventQueueIn, eventParamQueueIn, queueSize)
%#eml
% This function creates packets from the event queue. A packet consists
% of a destination, a message and an optional parameter for the message.
% Destination and message are contained at position 1 and 2 in the 
% eventQueue. Because of the different data type the parameter has his own 
% queue eventParamQueue.

%Constants
DESTINATION = 2;
MESSAGE = 1;
QUEUE_SIZE = queueSize;

busSize = numel(busSizeSignal);

%Init
eventQueue = eventQueueIn;
eventParamQueue = eventParamQueueIn;
packetMsg = zeros(1,busSize,'uint16');
packetParam = zeros(1,busSize,'double');

%There is an event in the queue
for i = 1:busSize   
    if eventQueue(1,DESTINATION) ~= 0 || eventQueue(1,MESSAGE) ~= 0
        %Create packet from the firs entry in the queue
        packetMsg(i)   = uint16(eventQueue(1,MESSAGE));
        packetParam(i) = eventParamQueue(1);
        %Remove the event from the queue
        for j=1:QUEUE_SIZE - 1
            eventQueue(j,DESTINATION)   = eventQueue(j+1,DESTINATION);
            eventQueue(j,MESSAGE)       = eventQueue(j+1,MESSAGE);
            eventParamQueue(j)          = eventParamQueue(j+1);
        end
        %Set last element to zero
        eventQueue(QUEUE_SIZE,DESTINATION)  = 0;
        eventQueue(QUEUE_SIZE,MESSAGE)      = 0;
        eventParamQueue(QUEUE_SIZE)    = 0;
    else
        break;
    end
end
